simulink subsystem "tire_model"  (R2019b)
settings: Solver=VariableStepAuto  StartTime=0.0  StopTime=10.0  RelTol=1e-3
libraries: simulink_extras x1
settings Model: Creator=yafta  LastModifiedBy=yafta

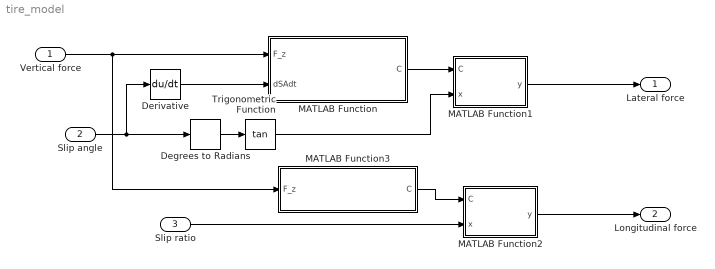
== system tire_model ==
  Vertical force : Inport
  Slip angle : Inport  Port=2
  Slip ratio : Inport  Port=3
  Degrees to Radians : simulink_extras/Transformations/Degrees to Radians
  Derivative : Derivative
  MATLAB Function : MATLAB Function  TreatAsAtomicUnit=on
  MATLAB Function1 : MATLAB Function  TreatAsAtomicUnit=on
  MATLAB Function2 : MATLAB Function  TreatAsAtomicUnit=on
  MATLAB Function3 : MATLAB Function  TreatAsAtomicUnit=on
  Trigonometric Function : Trigonometry  Operator=tan  OutputSignalType=real
  Lateral force : Outport
  Longitudinal force : Outport  Port=2
  wires:
  Slip angle/1 -> Degrees to Radians/1, Derivative/1
  MATLAB Function/1(C) -> MATLAB Function1/1(C)
  Trigonometric Function/1 -> MATLAB Function1/2(x)
  MATLAB Function1/1(y) -> Lateral force/1
  Derivative/1 -> MATLAB Function/2(dSAdt)
  Vertical force/1 -> MATLAB Function3/1(F_z), MATLAB Function/1(F_z)
  Degrees to Radians/1 -> Trigonometric Function/1
  MATLAB Function2/1(y) -> Longitudinal force/1
  MATLAB Function3/1(C) -> MATLAB Function2/1(C)
  Slip ratio/1 -> MATLAB Function2/2(x)

== matlab function tire_model/MATLAB Function1 ==
  data: C input; y output; x input
function y = pacejka(C,x)
y=C(3)*sin(C(2)*atan(C(1)*(1-C(4))*x+C(4)*atan(C(1)*x)));
end

== matlab function tire_model/MATLAB Function ==
  data: F_z input; dSAdt input; C output
function C = find_lat_coefficients(F_z,dSAdt)
[Ctotal]=load('pacejka_coefficients_lateral.mat');
n=0;
if F_z < -970
    n=0;
elseif F_z < -760
    n=2;
elseif F_z < -550
    n=4;
elseif F_z < -340
    n=8;
else
    n=6;
end
if dSAdt >= 0
    n=n+1;
end
C=Ctotal(n,:);
end

== matlab function tire_model/MATLAB Function2 ==
  data: C input; y output; x input
function y = pacejka(C,x)
y=C(3)*sin(C(2)*atan(C(1)*(1-C(4))*x+C(4)*atan(C(1)*x)));
end

== matlab function tire_model/MATLAB Function3 ==
  data: F_z input; C output
function C = find_long_coefficients(F_z)
[Ctotal]=load('pacejka_coefficients_longitudinal.mat');
n=0;
if F_z < -960
    n=1;
elseif F_z < -760
    n=2;
elseif F_z < -400
    n=3;
else
    n=5;
end
C=Ctotal(n,:);
end
